simulink model "First_Method"  (R2016b)
settings: Solver=VariableStepAuto  StartTime=0.0  StopTime=10.0  RelTol=1e-3
undefined symbols (not defined in the file): Be, D0, I0, Mx, My, Mz
settings Model: Creator=vbele  LastModifiedBy=vbele

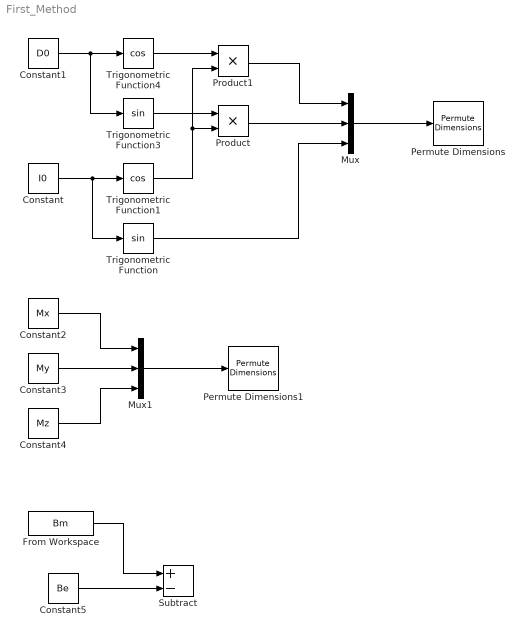
== system First_Method ==
  Constant : Constant  Value=I0
  Constant1 : Constant  Value=D0
  Constant2 : Constant  Value=Mx
  Constant3 : Constant  Value=My
  Constant4 : Constant  Value=Mz
  Constant5 : Constant  Value=Be
  From Workspace : FromWorkspace  VariableName=Bm  SampleTime=0
  Mux : Mux  Inputs=3
  Mux1 : Mux  Inputs=3
  Permute Dimensions : PermuteDimensions
  Permute Dimensions1 : PermuteDimensions
  Product : Product
  Product1 : Product
  Subtract : Sum  Inputs=+-
  Trigonometric Function : Trigonometry
  Trigonometric Function1 : Trigonometry  Operator=cos
  Trigonometric Function3 : Trigonometry
  Trigonometric Function4 : Trigonometry  Operator=cos
  wires:
  From Workspace/1 -> Subtract/1
  Constant1/1 -> Trigonometric Function4/1, Trigonometric Function3/1
  Constant/1 -> Trigonometric Function/1, Trigonometric Function1/1
  Trigonometric Function1/1 -> Product1/2, Product/2
  Trigonometric Function3/1 -> Product/1
  Trigonometric Function4/1 -> Product1/1
  Product1/1 -> Mux/1
  Product/1 -> Mux/2
  Trigonometric Function/1 -> Mux/3
  Constant2/1 -> Mux1/1
  Constant3/1 -> Mux1/2
  Constant4/1 -> Mux1/3
  Constant5/1 -> Subtract/2
  Mux/1 -> Permute Dimensions/1
  Mux1/1 -> Permute Dimensions1/1
